simulink model "Aero_Servo"  (R2014b)
settings: Solver=ode45  StartTime=tmin  StopTime=tmax  MaxStep=dt  RelTol=1e-3  AbsTol=1e-6
values from neighbouring files (symbols this model uses):
  dt = 0.001    [G3_Aero_Servo_Appdx.m]
  MCC = MM\CC    [G3_Aero_Servo_Appdx.m]
  MFG = MM\F_gust    [G3_Aero_Servo_Appdx.m]
  MKK = MM\KK    [G3_Aero_Servo_Appdx.m]
settings Model: Creator=User  LastModifiedBy=User
settings DataIOCC: SignalLoggingSaveFormat=ModelDataLogs  SignalLoggingName=sigsOut
settings OptimizationCC: InitFltsAndDblsToZero=on
settings DebuggingCC: SaveWithParameterizedLinksMsg=none  UnderspecifiedInitializationDetection=Classic  MergeDetectMultiDrivingBlocksExec=none  SignalResolutionControl=TryResolveAllWithWarning  SolverPrmCheckMsg=none  MultiTaskDSMMsg=warning  MultiTaskCondExecSysMsg=none  FcnCallInpInsideContextMsg=UseLocalSettings
settings HardwareCC: TargetUnknown=on
settings RTWCC: IncludeERTFirstTime=on
settings GRTTargetCC: TargetFcnLib=ansi_tfl_tmw.mat  ModelReferenceCompliant=off  CombineOutputUpdateFcns=off  MatFileLogging=off  GRTInterface=on

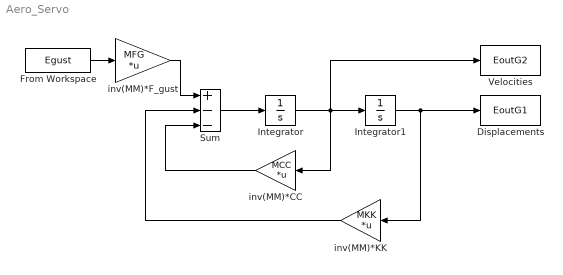
== system Aero_Servo ==
  Displacements : ToWorkspace  VariableName=EoutG1  SampleTime=dt
  From Workspace : FromWorkspace  VariableName=Egust  SampleTime=dt
  Integrator : Integrator
  Integrator1 : Integrator
  Sum : Sum  Inputs=+--  SaturateOnIntegerOverflow=on
  Velocities : ToWorkspace  VariableName=EoutG2  SampleTime=dt
  inv(MM)*CC : Gain  Gain=MCC  Multiplication=Matrix(K*u)  SaturateOnIntegerOverflow=on  OutDataTypeStr=Inherit: Same as input  ParamDataTypeStr=Inherit: Same as input
  inv(MM)*F_gust : Gain  Gain=MFG  Multiplication=Matrix(K*u) (u vector)  SaturateOnIntegerOverflow=on  OutDataTypeStr=Inherit: Same as input  ParamDataTypeStr=Inherit: Same as input
  inv(MM)*KK : Gain  Gain=MKK  Multiplication=Matrix(K*u)  SaturateOnIntegerOverflow=on  OutDataTypeStr=Inherit: Same as input  ParamDataTypeStr=Inherit: Same as input
  wires:
  Integrator/1 -> Integrator1/1, inv(MM)*CC/1, Velocities/1
  Sum/1 -> Integrator/1
  Integrator1/1 -> Displacements/1, inv(MM)*KK/1
  From Workspace/1 -> inv(MM)*F_gust/1
  inv(MM)*F_gust/1 -> Sum/1
  inv(MM)*CC/1 -> Sum/3
  inv(MM)*KK/1 -> Sum/2
